simulink model "Kalman_Unit_Step"  (R2023b)
settings: Solver=VariableStepAuto  StartTime=0.0  StopTime=20  RelTol=1e-3
undefined symbols (not defined in the file or in its folder): Discrete, Time
libraries: simulink x3, ctrlSharedLib x1
settings Model: Creator=sambr  LastModifiedBy=sambr

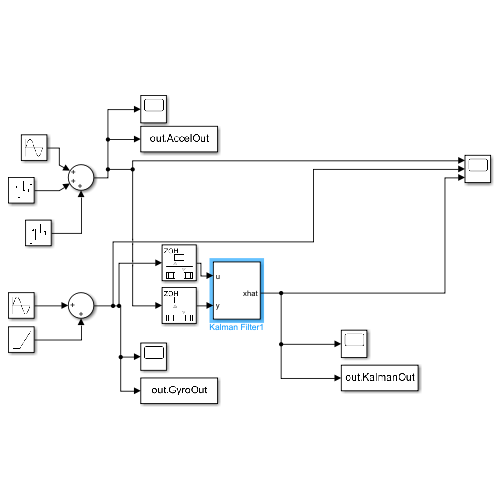
[thumbnail: Simulink's stored preview of the top-level diagram]
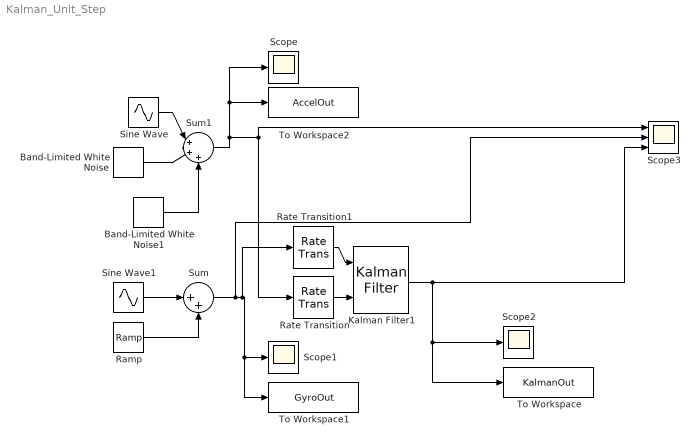
== system Kalman_Unit_Step ==
  Band-Limited White Noise : simulink/Sources/Band-Limited White Noise  Cov=[0.1]  Ts=0.01  seed=[23341]
  Band-Limited White Noise1 : simulink/Sources/Band-Limited White Noise  Cov=50  Ts=0.5  seed=[23341]
  Kalman Filter1 : ctrlSharedLib/Kalman Filter  TimeDomain=Discrete-Time  UseCurrentEstimator=on  ModelSource=Individual A, B, C, D matrices  ModelSourceVariable=ss(0.95,1,1,0,1)  A=0.95  B=0.02  C=0.05  D=0.001  NumberOfStates=1  NumberOfInputs=1  NumberOfOutputs=1  InitialEstimateSource=Dialog  X0=0  P0=10  UseK=off  UseGH=off  NumberOfProcessNoiseInputs=1  G=1  TimeInvariantG=on  H=0  TimeInvariantH=on  Q=0.01  TimeInvariantQ=on  R=2  TimeInvariantR=on  N=0  TimeInvariantN=on  AddInputPort=on  AddEnablePort=off  OutputEstimatedY=off  OutputP=off  Ts=0.001
  Ramp : simulink/Sources/Ramp  slope=2  start=0  InitialOutput=0
  Rate Transition : RateTransition  OutPortSampleTime=0.001
  Rate Transition1 : RateTransition  OutPortSampleTime=0.001
  Scope : Scope
  Scope1 : Scope
  Scope2 : Scope
  Scope3 : Scope  NumInputPorts=3
  Sine Wave : Sin  Amplitude=15  SampleTime=0
  Sine Wave1 : Sin  Amplitude=15  Bias=-5  SampleTime=0
  Sum : Sum  Inputs=|++
  Sum1 : Sum  Inputs=|+++
  To Workspace : ToWorkspace  VariableName=KalmanOut  SaveFormat=Structure With Time  SampleTime=-1
  To Workspace1 : ToWorkspace  VariableName=GyroOut  SaveFormat=Timeseries  SampleTime=-1
  To Workspace2 : ToWorkspace  VariableName=AccelOut  SaveFormat=Timeseries  SampleTime=-1
  wires:
  Kalman Filter1/1 -> To Workspace/1, Scope2/1, Scope3/3
  Sum1/1 -> To Workspace2/1, Scope/1, Rate Transition/1, Scope3/1
  Sum/1 -> Scope3/2, Rate Transition1/1, To Workspace1/1, Scope1/1
  Sine Wave1/1 -> Sum/1
  Sine Wave/1 -> Sum1/1
  Ramp/1 -> Sum/2
  Rate Transition/1 -> Kalman Filter1/2
  Rate Transition1/1 -> Kalman Filter1/1
  Band-Limited White Noise/1 -> Sum1/2
  Band-Limited White Noise1/1 -> Sum1/3
